simulink model "Copy_of_Qrotor_sim2"  (R2016a)
settings: Solver=ode4  StartTime=0.0  StopTime=T  FixedStep=0.001  RelTol=1e-3
values from neighbouring files (symbols this model uses):
  g = 9.81    [Sim_params.m]
  Ixx = 0.002100    (= 0.0021)    [Drone_params.m]
  Iyy = 0.002417    [Drone_params.m]
  Izz = 0.004633    [Drone_params.m]
  k_learn = 0.000001    (= 1e-06)    [Control_params.m]
  Ki = 3    [Control_params.m]
  KM_1 = KM_GENERAL    (= 0.00509)    [Drone_params.m]
  KM_2 = KM_GENERAL    (= 0.00509)    [Drone_params.m]
  KM_3 = KM_GENERAL    (= 0.00509)    [Drone_params.m]
  KM_4 = KM_GENERAL    (= 0.00509)    [Drone_params.m]
  KM_GENERAL = 0.00509    [Drone_params.m]
  KM_T_1 = KM_T_GENERAL    (= 5e-06)    [Drone_params.m]
  KM_T_2 = KM_T_GENERAL    (= 5e-06)    [Drone_params.m]
  KM_T_3 = KM_T_GENERAL    (= 5e-06)    [Drone_params.m]
  KM_T_4 = KM_T_GENERAL    (= 5e-06)    [Drone_params.m]
  KM_T_GENERAL = 0.000005    (= 5e-06)    [Drone_params.m]
  Kp = Ixx * Ki    [Control_params.m]
  KpP = 5    [Control_params.m]
  m = 0.475    [Drone_params.m]
  n_freq = 0.5    [Sim_params.m]
  PWM_CUT = 1000    [Drone_params.m]
  Tau_1 = Tau    (= 0.1)    [Drone_params.m]
  Tau_2 = Tau    (= 0.1)    [Drone_params.m]
  Tau_3 = Tau    (= 0.1)    [Drone_params.m]
  Tau_4 = Tau    (= 0.1)    [Drone_params.m]
  wnd_amp_p = .1    (= 0.1)    [Wind_params.m]
  wnd_amp_q = 0    [Wind_params.m]
  wnd_amp_r = 0    [Wind_params.m]
  wnd_amp_x = .1    (= 0.1)    [Wind_params.m]
  wnd_amp_y = .1    (= 0.1)    [Wind_params.m]
  wnd_amp_z = .1    (= 0.1)    [Wind_params.m]
  wnd_end_p = 20    [Wind_params.m]
  wnd_end_q = 15    [Wind_params.m]
  wnd_end_r = 15    [Wind_params.m]
  wnd_end_x = 44    [Wind_params.m]
  wnd_end_y = 31    [Wind_params.m]
  wnd_end_z = 49    [Wind_params.m]
  wnd_pqr_enable = 0    [Sim_params.m]
  wnd_ramp_p = 2*pi    (= 6.28318530718)    [Wind_params.m]
  wnd_ramp_q = 0.2    [Wind_params.m]
  wnd_ramp_r = 0.2    [Wind_params.m]
  wnd_ramp_x = .3    (= 0.3)    [Wind_params.m]
  wnd_ramp_y = .3    (= 0.3)    [Wind_params.m]
  wnd_ramp_z = .3    (= 0.3)    [Wind_params.m]
  wnd_start_p = 2    [Wind_params.m]
  wnd_start_q = 2    [Wind_params.m]
  wnd_start_r = 2    [Wind_params.m]
  wnd_start_x = 8    [Wind_params.m]
  wnd_start_y = 3    [Wind_params.m]
  wnd_start_z = 11    [Wind_params.m]
  wnd_xyz_enable = 0    [Sim_params.m]
  X_length = 0.155    [Drone_params.m]
  Y_length = 0.200    (= 0.2)    [Drone_params.m]
undefined symbols (not defined in the file or in its folder): X, Y, Z
libraries: simulink x12, sm_lib x10, nesl_utility x10
(part 1 of 2)
settings Model: Creator=Jet  LastModifiedBy=Jet

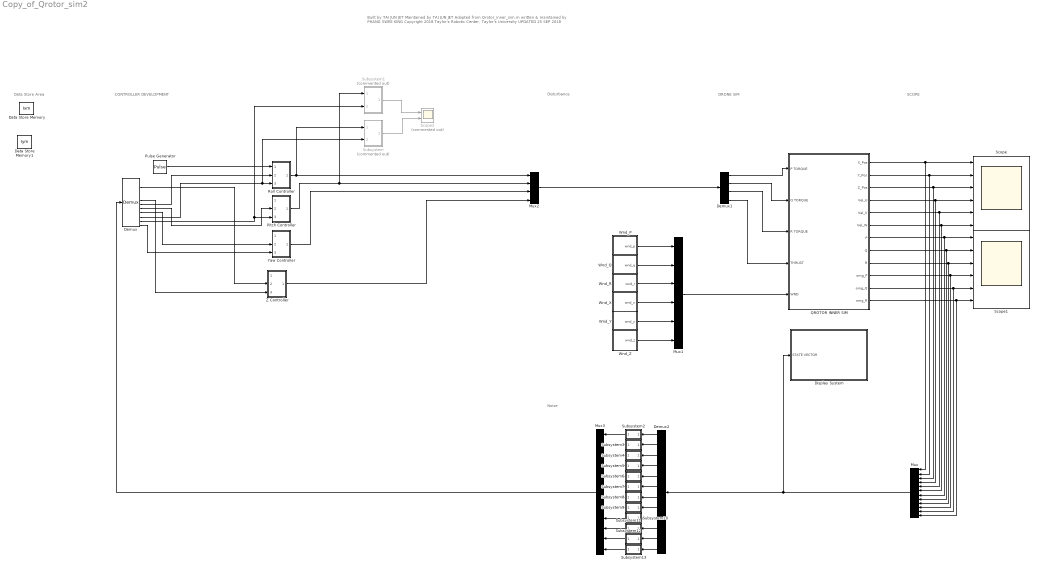
== system Copy_of_Qrotor_sim2 ==
  note: Noise
  note: Data Store Area
  note: Disturbance
  note: SCOPE
  note: DRONE SIM
  note: CONTROLLER DEVELOPMENT
  note: Built by TAI JUN JET
      | Maintained by TAI JUN JET
      | Adopted from Qrotor_inner_sim.m written & maintained by PHANG SWEE KING
      | Copyright 2018 Taylor's Robotic Center, Taylor's University
      | UPDATED 25 SEP 2018
  Data Store Memory : DataStoreMemory  DataStoreName=Ixm  ReadBeforeWriteMsg=warning  WriteAfterWriteMsg=warning  WriteAfterReadMsg=warning  InitialValue=Ixm  ShowAdditionalParam=off  OutDataTypeStr=double
  Data Store Memory1 : DataStoreMemory  DataStoreName=Iym  ReadBeforeWriteMsg=warning  WriteAfterWriteMsg=warning  WriteAfterReadMsg=warning  InitialValue=Iym  ShowAdditionalParam=off  OutDataTypeStr=double
  Demux : Demux  Outputs=12
  Demux1 : Demux
  Demux2 : Demux  Outputs=12
  Display System : Subsystem
  Mux : Mux  Inputs=12
  Mux1 : Mux  Inputs=6
  Mux2 : Mux
  Mux3 : Mux  Inputs=12
  Pitch Controller : Subsystem
  Pulse Generator : DiscretePulseGenerator  PulseType=Time based  Period=11  PulseWidth=50
  "QROTOR INNER SIM " : Subsystem
  "Roll Controller " : Subsystem
  Scope : Scope  NumInputPorts=6
  Scope1 : Scope  NumInputPorts=6
  Scope2 : Scope  Commented=on  NumInputPorts=2
  Subsystem : Subsystem  Commented=on
  Subsystem1 : Subsystem  Commented=on
  Subsystem10 : Subsystem
  Subsystem11 : Subsystem
  Subsystem12 : Subsystem
  Subsystem13 : Subsystem
  Subsystem2 : Subsystem
  Subsystem3 : Subsystem
  Subsystem4 : Subsystem
  Subsystem5 : Subsystem
  Subsystem6 : Subsystem
  Subsystem7 : Subsystem
  Subsystem8 : Subsystem
  Subsystem9 : Subsystem
  Wnd_P : Subsystem
  Wnd_Q : Subsystem
  Wnd_R : Subsystem
  Wnd_X : Subsystem
  Wnd_Y : Subsystem
  Wnd_Z : Subsystem
  Yaw Controller : Subsystem
  "Z Controller " : Subsystem
  wires:
  Mux/1 -> Display System/1(STATE VECTOR), Demux2/1
  Demux/10 -> Subsystem/2(In3), "Roll Controller "/3(In3)
  "QROTOR INNER SIM "/7(P) -> Scope1/1, Mux/7
  "QROTOR INNER SIM "/9(R) -> Scope1/3, Mux/9
  "QROTOR INNER SIM "/2(Y_Pos) -> Scope/2, Mux/2
  "QROTOR INNER SIM "/6(Vel_W) -> Scope/6, Mux/6
  "QROTOR INNER SIM "/11(omg_Q) -> Scope1/5, Mux/11
  "QROTOR INNER SIM "/12(omg_R) -> Scope1/6, Mux/12
  "QROTOR INNER SIM "/1(X_Pos) -> Scope/1, Mux/1
  "QROTOR INNER SIM "/10(omg_P) -> Scope1/4, Mux/10
  "QROTOR INNER SIM "/5(Vel_V) -> Scope/5, Mux/5
  "QROTOR INNER SIM "/8(Q) -> Scope1/2, Mux/8
  "QROTOR INNER SIM "/4(Vel_U) -> Scope/4, Mux/4
  "QROTOR INNER SIM "/3(Z_Pos) -> Scope/3, Mux/3
  Wnd_P/1(wnd_p) -> Mux1/1
  Wnd_Q/1(wnd_q) -> Mux1/2
  Wnd_R/1("wnd_r ") -> Mux1/3
  Wnd_X/1(wnd_x) -> Mux1/4
  Wnd_Y/1(wnd_y) -> Mux1/5
  Wnd_Z/1(wnd_z) -> Mux1/6
  "Roll Controller "/1(Out1) -> Subsystem/1(In2), Mux2/1
  Yaw Controller/1(Out1) -> Mux2/3
  Mux2/1 -> Demux1/1
  Demux1/1 -> "QROTOR INNER SIM "/1(P TORQUE)
  Demux1/2 -> "QROTOR INNER SIM "/2(Q TORQUE)
  Demux1/3 -> "QROTOR INNER SIM "/3(R TORQUE)
  Demux1/4 -> "QROTOR INNER SIM "/4(THRUST)
  Mux1/1 -> "QROTOR INNER SIM "/5(WND)
  Demux/3 -> "Z Controller "/2(In2)
  Demux/6 -> "Z Controller "/3(In3)
  "Z Controller "/1(Out1) -> Mux2/4
  Demux/11 -> Pitch Controller/3(In3), Subsystem1/2(In3)
  Pitch Controller/1(Out1) -> Subsystem1/1(In2), Mux2/2
  Subsystem1/1(Ixm) -> Scope2/1
  Subsystem/1(Iym) -> Scope2/2
  Pulse Generator/1 -> "Roll Controller "/1(In1)
  Demux/8 -> Pitch Controller/2(In2)
  Demux/9 -> Yaw Controller/2(In2)
  Demux/12 -> Yaw Controller/3(In3)
  Demux2/1 -> Subsystem2/1(In1)
  Demux2/2 -> Subsystem3/1(In1)
  Demux2/3 -> Subsystem4/1(In1)
  Demux2/4 -> Subsystem5/1(In1)
  Demux2/5 -> Subsystem6/1(In1)
  Demux2/6 -> Subsystem7/1(In1)
  Demux2/7 -> Subsystem8/1(In1)
  Demux2/8 -> Subsystem9/1(In1)
  Demux2/9 -> Subsystem10/1(In1)
  Demux2/10 -> Subsystem11/1(In1)
  Demux2/11 -> Subsystem12/1(In1)
  Demux2/12 -> Subsystem13/1(In1)
  Subsystem2/1(Out1) -> Mux3/1
  Subsystem3/1(Out1) -> Mux3/2
  Subsystem4/1(Out1) -> Mux3/3
  Subsystem5/1(Out1) -> Mux3/4
  Subsystem6/1(Out1) -> Mux3/5
  Subsystem7/1(Out1) -> Mux3/6
  Subsystem8/1(Out1) -> Mux3/7
  Subsystem9/1(Out1) -> Mux3/8
  Subsystem10/1(Out1) -> Mux3/9
  Subsystem11/1(Out1) -> Mux3/10
  Subsystem12/1(Out1) -> Mux3/11
  Subsystem13/1(Out1) -> Mux3/12
  Mux3/1 -> Demux/1
  Demux/7 -> "Roll Controller "/2(In2)

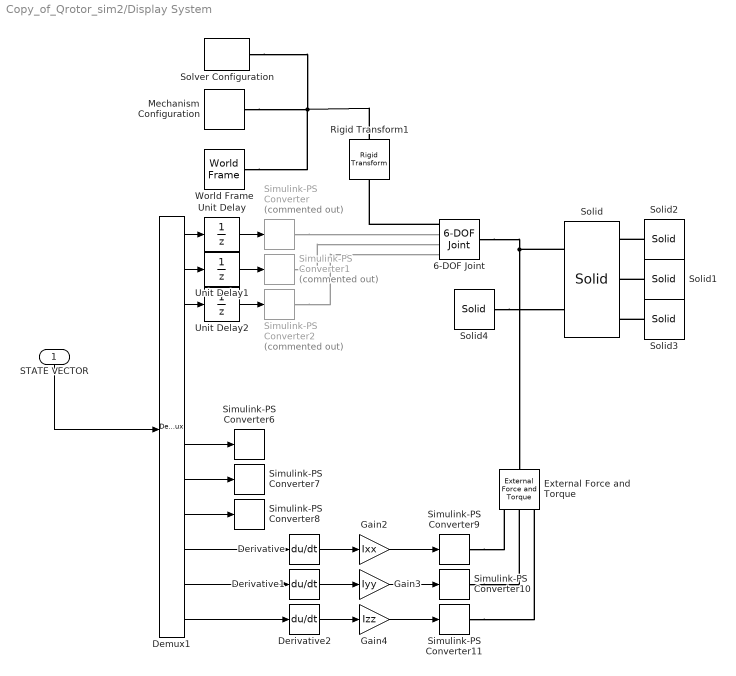
== system Copy_of_Qrotor_sim2/Display System ==
  STATE VECTOR : Inport
  6-DOF Joint : sm_lib/Joints/6-DOF Joint  SenseConstraintForce=off  SenseConstraintForceX=off  SenseConstraintForceY=off  SenseConstraintForceZ=off  SenseConstraintTorque=off  SenseConstraintTorqueX=off  SenseConstraintTorqueY=off  SenseConstraintTorqueZ=off  SenseTotalForce=off  SenseTotalForceX=off  SenseTotalForceY=off  SenseTotalForceZ=off  SenseTotalTorque=off  SenseTotalTorqueX=off  SenseTotalTorqueY=off  SenseTotalTorqueZ=off  CompositeWrenchDir=FollowerOnBase  CompositeWrenchFrame=BaseFrame  PxEquilibriumPosition=0  PxEquilibriumPositionUnits=m  PxSpringStiffness=0  PxSpringStiffnessUnits=N/m  PxDampingCoefficient=0  PxDampingCoefficientUnits=N/(m/s)  PxTorqueActuationMode=ComputedTorque  PxMotionActuationMode=InputMotion  PxSensePosition=off  PxSenseVelocity=off  PxSenseAcceleration=off  PxSenseTorqueForce=off  PxPositionTargetSpecify=on  PxPositionTargetPriority=High  PxPositionTargetValue=0  PxPositionTargetValueUnits=m  PxVelocityTargetSpecify=on  PxVelocityTargetPriority=High  PxVelocityTargetValue=0  PxVelocityTargetValueUnits=m/s  PyEquilibriumPosition=0  PyEquilibriumPositionUnits=m  PySpringStiffness=0  PySpringStiffnessUnits=N/m  PyDampingCoefficient=0  PyDampingCoefficientUnits=N/(m/s)  PyTorqueActuationMode=ComputedTorque  PyMotionActuationMode=InputMotion  PySensePosition=off  PySenseVelocity=off  PySenseAcceleration=off  PySenseTorqueForce=off  PyPositionTargetSpecify=on  PyPositionTargetPriority=High  PyPositionTargetValue=0  PyPositionTargetValueUnits=m  PyVelocityTargetSpecify=on  PyVelocityTargetPriority=High  PyVelocityTargetValue=0  PyVelocityTargetValueUnits=m/s  PzEquilibriumPosition=0  PzEquilibriumPositionUnits=m  PzSpringStiffness=0  PzSpringStiffnessUnits=N/m  PzDampingCoefficient=0  PzDampingCoefficientUnits=N/(m/s)  PzTorqueActuationMode=ComputedTorque  PzMotionActuationMode=InputMotion  PzSensePosition=off  PzSenseVelocity=off  PzSenseAcceleration=off  PzSenseTorqueForce=off  PzPositionTargetSpecify=on  PzPositionTargetPriority=High  PzPositionTargetValue=0  PzPositionTargetValueUnits=m  PzVelocityTargetSpecify=on  PzVelocityTargetPriority=High  PzVelocityTargetValue=0  PzVelocityTargetValueUnits=m/s  SphDefPosRotationMethod=None  SphDefPosRotationAngleUnits=deg  SphDefPosRotationStandardAxis=+Z  SphDefPosRotationAngle=0.0  SphDefPosRotationArbitraryAxis=[0 0 1]  SphDefPosFollAlignAxisA=+X  SphDefPosBaseAlignAxisA=+Y  SphDefPosFollAlignAxisB=+Y  SphDefPosBaseAlignAxisB=+Z  SphDefPosRotationSequenceAxes=FollowerAxes  SphDefPosRotationSequence=XYX  SphDefPosRotationSequenceAngles=[0 0 0]  SphDefPosRotationSequenceAnglesUnits=deg  SphDefPosRotationMatrix=[1 0 0; 0 1 0; 0 0 1]  SphEqPosRotationMethod=None  SphEqPosRotationAngleUnits=deg  SphEqPosRotationStandardAxis=+Z  SphEqPosRotationAngle=0.0  SphEqPosRotationArbitraryAxis=[0 0 1]  SphEqPosFollAlignAxisA=+X  SphEqPosBaseAlignAxisA=+Y  SphEqPosFollAlignAxisB=+Y  SphEqPosBaseAlignAxisB=+Z  SphEqPosRotationSequenceAxes=FollowerAxes  SphEqPosRotationSequence=XYX  SphEqPosRotationSequenceAngles=[0 0 0]  SphEqPosRotationSequenceAnglesUnits=deg  SphEqPosRotationMatrix=[1 0 0; 0 1 0; 0 0 1]  SphSpringStiffness=0  SphSpringStiffnessUnits=N*m/deg  SphDampingCoefficient=0  SphDampingCoefficientUnits=N*m/(deg/s)  SphActuateTorqueX=off  SphActuateTorqueY=off  SphActuateTorqueZ=off  SphActuateTorque=off  SphTorqueActuationMode=NoTorque  SphMotionActuationMode=ComputedMotion  SphActuationFrame=BaseFrame  SphSensePosition=off  SphSenseVelocityX=off  SphSenseVelocityY=off  SphSenseVelocityZ=off  SphSenseVelocity=off  SphSenseAccelerationX=off  SphSenseAccelerationY=off  SphSenseAccelerationZ=off  SphSenseAcceleration=off  SphSenseTorqueX=off  SphSenseTorqueY=off  SphSenseTorqueZ=off  SphSenseTorqueForce=off  SphSensingFrame=BaseFrame  SphPositionTargetRotationMethod=None  SphPositionTargetRotationAngleUnits=deg  SphPositionTargetRotationStandardAxis=+Z  SphPositionTargetRotationAngle=0.0  SphPositionTargetRotationArbitraryAxis=[0 0 1]  SphPositionTargetFollAlignAxisA=+X  SphPositionTargetBaseAlignAxisA=+Y  SphPositionTargetFollAlignAxisB=+Y  SphPositionTargetBaseAlignAxisB=+Z  SphPositionTargetRotationSequenceAxes=FollowerAxes  SphPositionTargetRotationSequence=XYX  SphPositionTargetRotationSequenceAngles=[0 0 0]  SphPositionTargetRotationSequenceAnglesUnits=deg  SphPositionTargetRotationMatrix=[1 0 0; 0 1 0; 0 0 1]  SphPositionTargetSpecify=off  SphPositionTargetPriority=High  SphVelocityTargetValue=[0 0 0]  SphVelocityTargetValueUnits=deg/s  SphVelocityTargetSpecify=off  SphVelocityTargetPriority=High  SphVelocityTargetInFollowerFrame=on
  Demux1 : Demux  Outputs=12
  Derivative : Derivative
  Derivative1 : Derivative
  Derivative2 : Derivative
  External Force and Torque : sm_lib/Forces and Torques/External Force and Torque  ForceResolutionFrame=AttachedFrame  EnableForceX=off  EnableForceY=off  EnableForceZ=off  EnableForce=off  TorqueResolutionFrame=AttachedFrame  EnableTorqueX=on  EnableTorqueY=on  EnableTorqueZ=on  EnableTorque=off
  Gain2 : Gain  Gain=Ixx
  Gain3 : Gain  Gain=Iyy
  Gain4 : Gain  Gain=Izz
  Mechanism Configuration : sm_lib/Utilities/Mechanism Configuration  UniformGravity=Constant  GravityVector=[0 0 0]  GravityUnits=m/s^2  LinearizationDelta=0.001
  Rigid Transform1 : sm_lib/Frames and Transforms/Rigid Transform  TranslationMethod=None  TranslationLengthUnit=m  TranslationStandardAxis=+Z  TranslationStandardOffset=0  TranslationCartesianOffset=[0 0 0]  TranslationROffset=0  TranslationROffsetUnits=m  TranslationZOffset=0  TranslationZOffsetUnits=m  TranslationThetaOffset=0  TranslationThetaOffsetUnits=deg  RotationMethod=AlignedAxes  RotationAngleUnits=deg  RotationStandardAxis=+Z  RotationAngle=0.0  RotationArbitraryAxis=[0 0 1]  FollAlignAxisA=+X  BaseAlignAxisA=+X  FollAlignAxisB=-Z  BaseAlignAxisB=+Z  RotationSequenceAxes=FollowerAxes  RotationSequence=XYX  RotationSequenceAngles=[0 0 0]  RotationSequenceAnglesUnits=deg  RotationMatrix=[1 0 0; 0 1 0; 0 0 1]
  Simulink-PS Converter : nesl_utility/Simulink-PS Converter  Commented=on  PhysicalDomain=network_engine_domain  SubClassName=ps_input  LeftPortType=input  RightPortType=output  PseudoPeriodic=off  Frequencies=[]  NoiseDistribution=none  NoiseParameters=[]  Unit=1  AffineConversion=off  InputFiltering=off  SimscapeFilterOrder=2  InputFilterTimeConstant=0.001  UdotUserProvided=1
  Simulink-PS Converter1 : nesl_utility/Simulink-PS Converter  Commented=on  PhysicalDomain=network_engine_domain  SubClassName=ps_input  LeftPortType=input  RightPortType=output  PseudoPeriodic=off  Frequencies=[]  NoiseDistribution=none  NoiseParameters=[]  Unit=1  AffineConversion=off  InputFiltering=off  SimscapeFilterOrder=2  InputFilterTimeConstant=0.001  UdotUserProvided=1
  Simulink-PS Converter{6..11} (6 alike) : nesl_utility/Simulink-PS Converter  PhysicalDomain=network_engine_domain  SubClassName=ps_input  LeftPortType=input  RightPortType=output  PseudoPeriodic=off  Frequencies=[]  NoiseDistribution=none  NoiseParameters=[]  Unit=1  AffineConversion=off  InputFiltering=off  SimscapeFilterOrder=1  InputFilterTimeConstant=0.001  UdotUserProvided=1
  Simulink-PS Converter2 : nesl_utility/Simulink-PS Converter  Commented=on  PhysicalDomain=network_engine_domain  SubClassName=ps_input  LeftPortType=input  RightPortType=output  PseudoPeriodic=off  Frequencies=[]  NoiseDistribution=none  NoiseParameters=[]  Unit=1  AffineConversion=off  InputFiltering=off  SimscapeFilterOrder=2  InputFilterTimeConstant=0.001  UdotUserProvided=1
  Solid : sm_lib/Body Elements/Solid  InertiaType=Custom  Mass=1  MassUnits=kg  CenterOfMass=[0 0 0]  CenterOfMassUnits=m  MomentsOfInertia=[Ixx Iyy Izz]  MomentsOfInertiaUnits=kg*m^2  ProductsOfInertia=[0 0 0]  ProductsOfInertiaUnits=kg*m^2  DensityBased=on  Density=1000  DensityUnits=kg/(m^3)  DoExposeReferenceFrame=on  SerializedFrames=<Frames><Frame><Id>Frame1</Id><Value><Name>F1</Name><Origin><Source>GeometricFeature</Source><FeatureName>+x -y -z point</FeatureName></Origin><PrimaryAxis><DefinedDirection>+Z</DefinedDirection><Source>ReferenceFrame</Source><SourceDirection>+Z</SourceDirection><FeatureName></FeatureName></PrimaryAxis><SecondaryAxis><DefinedDirection>+X</DefinedDirection><Source>ReferenceFrame</Source><SourceDirection>+X</SourceDirection><FeatureName></FeatureName></SecondaryAxis></Value></Frame><Frame><Id>Frame2</Id><Value><Name>F2</Name><Origin><Source>GeometricFeature</Source><FeatureName>+x +y -z point</FeatureName></Origin><PrimaryAxis><DefinedDirection>+Z</DefinedDirection><Source>ReferenceFrame</Source><SourceDirection>+Z</SourceDirection><FeatureName></FeatureName></PrimaryAxis><SecondaryAxis><DefinedDirection>+X</DefinedDirection><Source>ReferenceFrame</Source><SourceDirection>+X</SourceDirection><FeatureName></FeatureName></SecondaryAxis></Value></Frame><Frame><Id>Frame3</Id><Value><Name>F3</Name><Origin><Source>GeometricFeature</Source><FeatureName>-x -y -z point</FeatureName></Origin><PrimaryAxis><DefinedDirection>+Z</DefinedDirection><Source>ReferenceFrame</Source><SourceDirection>+Z</SourceDirection><FeatureName></FeatureName></PrimaryAxis><SecondaryAxis><DefinedDirection>+X</DefinedDirection><Source>ReferenceFrame</Source><SourceDirection>+X</SourceDirection><FeatureName></FeatureName></SecondaryAxis></Value></Frame><Frame><Id>Frame4</Id><Value><Name>F4</Name><Origin><Source>GeometricFeature</Source><FeatureName>-x +y -z point</FeatureName></Origin><PrimaryAxis><DefinedDirection>+Z</DefinedDirection><Source>ReferenceFrame</Source><SourceDirection>+Z</SourceDirection><FeatureName></FeatureName></PrimaryAxis><SecondaryAxis><DefinedDirection>+X</DefinedDirection><Source>ReferenceFrame</Source><SourceDirection>+X</SourceDirection><FeatureName></FeatureName></SecondaryAxis></Value></Frame></Frames>  GraphicType=FromGeometry  MarkerShape=Sphere  MarkerSize=10  GraphicVisPropType=SimpleVisualProperties  GraphicDiffuseColor=[1 0 0]  GraphicSpecularColor=[1 0.2 0 1.0]  GraphicAmbientColor=[1 .2 0 1.0]  GraphicEmissiveColor=[1 0.0 0.0 1.0]  GraphicShininess=0  GraphicOpacity=1  GeometryShape=Brick  RectangleSize=[1 1]  RectangleSizeUnits=m  BrickDimensions=[Y_length X_length X_length/3]  BrickDimensionUnits=m  CylinderRadius=1  CylinderRadiusUnits=m  CylinderLength=1  CylinderLengthUnits=m  SphereRadius=1  SphereRadiusUnits=m  EllipsoidRadii=[1 1 1]  EllipsoidRadiiUnits=m  ExtrusionCrossSection=[1 1; -1 1; -1 -1; 1 -1]  ExtrusionCrossSectionUnits=m  ExtrusionLength=1  ExtrusionLengthUnits=m  PolygonNumSides=3  PolygonOuterRadius=1  PolygonOuterRadiusUnits=m  ExtGeomFileType=STEP  ExtGeomFileUnits=m  RevolutionCrossSection=[1 1; 1 -1; 2 -1; 2 1]  RevolutionCrossSectionUnits=m  RevolutionExtent=Full  RevolutionAngle=180  RevolutionAngleUnits=deg
  Solid{1..4} (4 alike) : sm_lib/Body Elements/Solid  InertiaType=CalculateFromGeometry  Mass=1  MassUnits=kg  CenterOfMass=[0 0 0]  CenterOfMassUnits=m  MomentsOfInertia=[1 1 1]  MomentsOfInertiaUnits=kg*m^2  ProductsOfInertia=[0 0 0]  ProductsOfInertiaUnits=kg*m^2  DensityBased=on  Density=0  DensityUnits=kg/(m^3)  DoExposeReferenceFrame=on  SerializedFrames=<Frames/>  GraphicType=FromGeometry  MarkerShape=Sphere  MarkerSize=10  GraphicVisPropType=SimpleVisualProperties  GraphicDiffuseColor=[0.5 0.5 0.5]  GraphicSpecularColor=[0.5 0.5 0.5 1.0]  GraphicAmbientColor=[0.15 0.15 0.15 1.0]  GraphicEmissiveColor=[0.0 0.0 0.0 1.0]  GraphicShininess=75  GraphicOpacity=.2  GeometryShape=Cylinder  RectangleSize=[1 1]  RectangleSizeUnits=m  BrickDimensions=[.1 .1 .1]  BrickDimensionUnits=m  CylinderRadius=X_length*Y_length*2  CylinderRadiusUnits=m  CylinderLength=X_length*0.02  CylinderLengthUnits=m  SphereRadius=1  SphereRadiusUnits=m  EllipsoidRadii=[1 1 1]  EllipsoidRadiiUnits=m  ExtrusionCrossSection=[1 1; -1 1; -1 -1; 1 -1]  ExtrusionCrossSectionUnits=m  ExtrusionLength=1  ExtrusionLengthUnits=m  PolygonNumSides=3  PolygonOuterRadius=1  PolygonOuterRadiusUnits=m  ExtGeomFileType=STEP  ExtGeomFileUnits=m  RevolutionCrossSection=[1 1; 1 -1; 2 -1; 2 1]  RevolutionCrossSectionUnits=m  RevolutionExtent=Full  RevolutionAngle=180  RevolutionAngleUnits=deg
  Solver Configuration : nesl_utility/Solver Configuration  PhysicalDomain=network_engine_domain  SubClassName=solver  LeftPortType=input  RightPortType=generic  Accelerate=off  Tones=[]  Harmonics=[]  SimulateNoise=off  Profile=off  UseLocalSampling=off  EnableSwitchedLinearOptims=on  FrequencyDomain=off  UseCCode=off  RelTol=0.001  AbsTol=1e-06  MinStep=1e-09  ToWorkspace=off  RevertToSquareIcSolve=off  NumHomotopyIterations=100  PhasorMode=off  PhasorModeNumHarmonics=1  OverrideAbsTol=off  DoDC=off  ResidualTolerance=1e-09  UseLocalSolver=off  LocalSolverChoice=NE_BACKWARD_EULER_ADVANCER  LocalSolverSampleTime=0.001  DoFixedCost=off  MaxNonlinIter=3  MaxModeIter=2  LinearAlgebra=Sparse  DelaysMemoryBudget=1024  AutomaticFiltering=on  FilteringTimeConstant=0.001
  Unit Delay : UnitDelay  SampleTime=-1
  Unit Delay1 : UnitDelay  SampleTime=-1
  Unit Delay2 : UnitDelay  SampleTime=-1
  World Frame : sm_lib/Frames and Transforms/World Frame
  wires:
  Demux1/2 -> Unit Delay1/1
  Demux1/1 -> Unit Delay/1
  Demux1/3 -> Unit Delay2/1
  Demux1/7 -> Simulink-PS Converter6/1
  Demux1/8 -> Simulink-PS Converter7/1
  Unit Delay/1 -> Simulink-PS Converter/1
  Demux1/12 -> Derivative2/1
  Demux1/10 -> Derivative/1
  Derivative2/1 -> Gain4/1
  Derivative/1 -> Gain2/1
  Demux1/11 -> Derivative1/1
  Unit Delay2/1 -> Simulink-PS Converter2/1
  Gain2/1 -> Simulink-PS Converter9/1
  Gain4/1 -> Simulink-PS Converter11/1
  Demux1/9 -> Simulink-PS Converter8/1
  Derivative1/1 -> Gain3/1
  Gain3/1 -> Simulink-PS Converter10/1
  Unit Delay1/1 -> Simulink-PS Converter1/1
  STATE VECTOR/1 -> Demux1/1
  connections:
  Solid4/RConn1 -- Solid/RConn2
  Simulink-PS Converter1/RConn1 -- 6-DOF Joint/LConn3
  Simulink-PS Converter9/RConn1 -- External Force and Torque/LConn1
  Simulink-PS Converter2/RConn1 -- 6-DOF Joint/LConn4
  Simulink-PS Converter/RConn1 -- 6-DOF Joint/LConn2
  World Frame/RConn1 -- Rigid Transform1/LConn1 -- Mechanism Configuration/RConn1 -- Solver Configuration/RConn1
  Simulink-PS Converter10/RConn1 -- External Force and Torque/LConn2
  Simulink-PS Converter11/RConn1 -- External Force and Torque/LConn3
  Solid2/RConn1 -- Solid/LConn1
  Solid1/RConn1 -- Solid/LConn2
  Solid3/RConn1 -- Solid/LConn3
  Solid/RConn1 -- 6-DOF Joint/RConn1 -- External Force and Torque/RConn1
  6-DOF Joint/LConn1 -- Rigid Transform1/RConn1

== system Copy_of_Qrotor_sim2/Pitch Controller ==
  In1 : Inport
  In2 : Inport  Port=2
  In3 : Inport  Port=3
  Data Store Read : DataStoreRead  DataStoreName=Ixm
  Gain : Gain  Gain=KpP
  Integrator6 : Integrator
  K1 : Gain  Gain=Ki*Kp
  K2 : Gain  Gain=Ki
  Kp : Gain  Gain=Kp
  Matrix Multiply : Product  Multiplication=Matrix(*)
  Sum : Sum  Inputs=+-
  Sum1 : Sum  Inputs=+-
  Sum2 : Sum  Inputs=++-
  Out1 : Outport
  wires:
  K1/1 -> Integrator6/1
  Sum/1 -> K1/1, Kp/1
  In2/1 -> Sum1/2
  In3/1 -> Sum/2, K2/1
  In1/1 -> Sum1/1
  Sum2/1 -> Out1/1
  Integrator6/1 -> Sum2/1
  Kp/1 -> Sum2/2
  K2/1 -> Matrix Multiply/1
  Matrix Multiply/1 -> Sum2/3
  Data Store Read/1 -> Matrix Multiply/2
  Sum1/1 -> Gain/1
  Gain/1 -> Sum/1

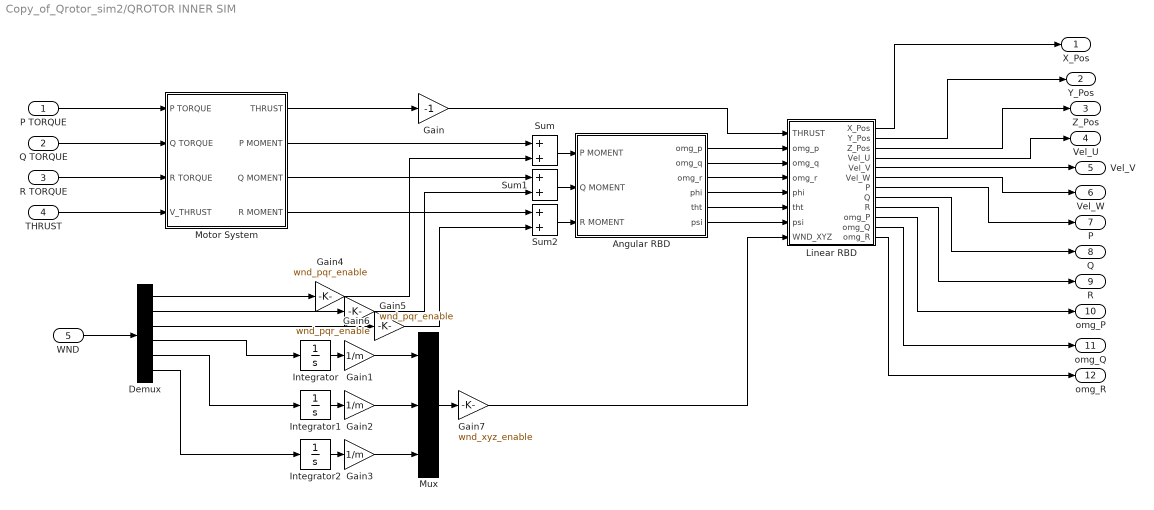
== system Copy_of_Qrotor_sim2/QROTOR INNER SIM  ==
  P TORQUE : Inport
  Q TORQUE : Inport  Port=2
  R TORQUE : Inport  Port=3
  THRUST : Inport  Port=4
  WND : Inport  Port=5
  Angular RBD : Subsystem
  Demux : Demux  Outputs=6
  Gain : Gain  Gain=-1
  Gain1 : Gain  Gain=1/m
  Gain2 : Gain  Gain=1/m
  Gain3 : Gain  Gain=1/m
  Gain4 : Gain  Gain=wnd_pqr_enable
  Gain5 : Gain  Gain=wnd_pqr_enable
  Gain6 : Gain  Gain=wnd_pqr_enable
  Gain7 : Gain  Gain=wnd_xyz_enable
  Integrator : Integrator
  Integrator1 : Integrator
  Integrator2 : Integrator
  Linear RBD : Subsystem
  "Motor System " : Subsystem
  Mux : Mux  Inputs=3
  Sum : Sum
  Sum1 : Sum
  Sum2 : Sum
  X_Pos : Outport
  Y_Pos : Outport  Port=2
  Z_Pos : Outport  Port=3
  Vel_U : Outport  Port=4
  Vel_V : Outport  Port=5
  Vel_W : Outport  Port=6
  P : Outport  Port=7
  Q : Outport  Port=8
  R : Outport  Port=9
  omg_P : Outport  Port=10
  omg_Q : Outport  Port=11
  omg_R : Outport  Port=12
  wires:
  Linear RBD/4(Vel_U) -> Vel_U/1
  Linear RBD/3(Z_Pos) -> Z_Pos/1
  Linear RBD/9(R) -> R/1
  Linear RBD/6(Vel_W) -> Vel_W/1
  Linear RBD/1(X_Pos) -> X_Pos/1
  Linear RBD/7(P) -> P/1
  Linear RBD/2(Y_Pos) -> Y_Pos/1
  Linear RBD/10(omg_P) -> omg_P/1
  Linear RBD/11(omg_Q) -> omg_Q/1
  Linear RBD/12(omg_R) -> omg_R/1
  Linear RBD/8(Q) -> Q/1
  Linear RBD/5(Vel_V) -> Vel_V/1
  Angular RBD/2(omg_q) -> Linear RBD/3(omg_q)
  Angular RBD/4(phi) -> Linear RBD/5(phi)
  Angular RBD/5(tht) -> Linear RBD/6(tht)
  Angular RBD/3(omg_r) -> Linear RBD/4(omg_r)
  Gain/1 -> Linear RBD/1(THRUST)
  Angular RBD/1(omg_p) -> Linear RBD/2(omg_p)
  Angular RBD/6(psi) -> Linear RBD/7(psi)
  THRUST/1 -> "Motor System "/4(V_THRUST)
  P TORQUE/1 -> "Motor System "/1(P TORQUE)
  R TORQUE/1 -> "Motor System "/3(R TORQUE)
  Q TORQUE/1 -> "Motor System "/2(Q TORQUE)
  Sum/1 -> Angular RBD/1(P MOMENT)
  Sum1/1 -> Angular RBD/2(Q MOMENT)
  Sum2/1 -> Angular RBD/3(R MOMENT)
  "Motor System "/2(P MOMENT) -> Sum/1
  "Motor System "/3(Q MOMENT) -> Sum1/1
  "Motor System "/4(R MOMENT) -> Sum2/1
  WND/1 -> Demux/1
  Demux/1 -> Gain4/1
  Demux/2 -> Gain5/1
  Demux/3 -> Gain6/1
  Integrator/1 -> Gain1/1
  Demux/4 -> Integrator/1
  Integrator1/1 -> Gain2/1
  Integrator2/1 -> Gain3/1
  Demux/5 -> Integrator1/1
  Demux/6 -> Integrator2/1
  Gain2/1 -> Mux/2
  Gain1/1 -> Mux/1
  Gain3/1 -> Mux/3
  Mux/1 -> Gain7/1
  Gain4/1 -> Sum/2
  Gain5/1 -> Sum1/2
  Gain6/1 -> Sum2/2
  Gain7/1 -> Linear RBD/8(WND_XYZ)
  "Motor System "/1(THRUST) -> Gain/1

== system Copy_of_Qrotor_sim2/Roll Controller  ==
  In1 : Inport
  In2 : Inport  Port=2
  In3 : Inport  Port=3
  Data Store Read : DataStoreRead  DataStoreName=Ixm
  Gain : Gain  Gain=KpP
  Integrator6 : Integrator
  K1 : Gain  Gain=Ki*Kp
  K2 : Gain  Gain=Ki
  Kp : Gain  Gain=Kp
  Matrix Multiply : Product  Multiplication=Matrix(*)
  Sum : Sum  Inputs=+-
  Sum1 : Sum  Inputs=+-
  Sum2 : Sum  Inputs=++-
  Out1 : Outport
  wires:
  K1/1 -> Integrator6/1
  Sum/1 -> K1/1, Kp/1
  In2/1 -> Sum1/2
  In3/1 -> Sum/2, K2/1
  In1/1 -> Sum1/1
  Sum2/1 -> Out1/1
  Integrator6/1 -> Sum2/1
  Kp/1 -> Sum2/2
  K2/1 -> Matrix Multiply/1
  Matrix Multiply/1 -> Sum2/3
  Data Store Read/1 -> Matrix Multiply/2
  Sum1/1 -> Gain/1
  Gain/1 -> Sum/1

== system Copy_of_Qrotor_sim2/Subsystem ==
  In2 : Inport
  In3 : Inport  Port=2
  Constant : Constant  Value=k_learn
  Data Store Read : DataStoreRead  DataStoreName=Iym
  Data Store Write : DataStoreWrite  DataStoreName=Iym
  Derivative1 : Derivative
  Iym Predictor : MATLAB Function  TreatAsAtomicUnit=on
  Iym : Outport
  wires:
  Data Store Read/1 -> Iym Predictor/4(Iym_sim)
  Iym Predictor/1(Iym_sim_out) -> Iym/1, Data Store Write/1
  Derivative1/1 -> Iym Predictor/1(domg_P)
  In3/1 -> Derivative1/1
  In2/1 -> Iym Predictor/2(p_torque)
  Constant/1 -> Iym Predictor/3(k_learn)

== system Copy_of_Qrotor_sim2/Subsystem1 ==
  In2 : Inport
  In3 : Inport  Port=2
  Constant : Constant  Value=k_learn
  Data Store Read : DataStoreRead  DataStoreName=Ixm
  Data Store Write : DataStoreWrite  DataStoreName=Ixm
  Derivative1 : Derivative
  Ixm Predictor : MATLAB Function  TreatAsAtomicUnit=on
  Ixm : Outport
  wires:
  Data Store Read/1 -> Ixm Predictor/4(Ixm_sim)
  Derivative1/1 -> Ixm Predictor/1(domg_P)
  In3/1 -> Derivative1/1
  In2/1 -> Ixm Predictor/2(p_torque)
  Constant/1 -> Ixm Predictor/3(k_learn)
  Ixm Predictor/1(Ixm_sim_out) -> Ixm/1, Data Store Write/1

== system Copy_of_Qrotor_sim2/Subsystem10 ==
  In1 : Inport
  Band-Limited White Noise : simulink/Sources/Band-Limited White Noise  Cov=n_power  Ts=n_freq  seed=[23341]
  Rate Transition : RateTransition
  Sum : Sum
  Out1 : Outport
  wires:
  Sum/1 -> Out1/1
  In1/1 -> Sum/2
  Band-Limited White Noise/1 -> Rate Transition/1
  Rate Transition/1 -> Sum/1

== system Copy_of_Qrotor_sim2/Subsystem11 ==
  In1 : Inport
  Band-Limited White Noise : simulink/Sources/Band-Limited White Noise  Cov=n_power  Ts=n_freq  seed=[23341]
  Rate Transition : RateTransition
  Sum : Sum
  Out1 : Outport
  wires:
  Sum/1 -> Out1/1
  In1/1 -> Sum/2
  Band-Limited White Noise/1 -> Rate Transition/1
  Rate Transition/1 -> Sum/1

== system Copy_of_Qrotor_sim2/Subsystem12 ==
  In1 : Inport
  Band-Limited White Noise : simulink/Sources/Band-Limited White Noise  Cov=n_power  Ts=n_freq  seed=[23341]
  Rate Transition : RateTransition
  Sum : Sum
  Out1 : Outport
  wires:
  Sum/1 -> Out1/1
  In1/1 -> Sum/2
  Band-Limited White Noise/1 -> Rate Transition/1
  Rate Transition/1 -> Sum/1

== system Copy_of_Qrotor_sim2/Subsystem13 ==
  In1 : Inport
  Band-Limited White Noise : simulink/Sources/Band-Limited White Noise  Cov=n_power  Ts=n_freq  seed=[23341]
  Rate Transition : RateTransition
  Sum : Sum
  Out1 : Outport
  wires:
  Sum/1 -> Out1/1
  In1/1 -> Sum/2
  Band-Limited White Noise/1 -> Rate Transition/1
  Rate Transition/1 -> Sum/1

== system Copy_of_Qrotor_sim2/Subsystem2 ==
  In1 : Inport
  Band-Limited White Noise : simulink/Sources/Band-Limited White Noise  Cov=n_power  Ts=n_freq  seed=[23341]
  Rate Transition : RateTransition
  Sum : Sum
  Out1 : Outport
  wires:
  Sum/1 -> Out1/1
  In1/1 -> Sum/2
  Band-Limited White Noise/1 -> Rate Transition/1
  Rate Transition/1 -> Sum/1

== system Copy_of_Qrotor_sim2/Subsystem3 ==
  In1 : Inport
  Band-Limited White Noise : simulink/Sources/Band-Limited White Noise  Cov=n_power  Ts=n_freq  seed=[23341]
  Rate Transition : RateTransition
  Sum : Sum
  Out1 : Outport
  wires:
  Sum/1 -> Out1/1
  In1/1 -> Sum/2
  Band-Limited White Noise/1 -> Rate Transition/1
  Rate Transition/1 -> Sum/1

== system Copy_of_Qrotor_sim2/Subsystem4 ==
  In1 : Inport
  Band-Limited White Noise : simulink/Sources/Band-Limited White Noise  Cov=n_power  Ts=n_freq  seed=[23341]
  Rate Transition : RateTransition
  Sum : Sum
  Out1 : Outport
  wires:
  Sum/1 -> Out1/1
  In1/1 -> Sum/2
  Band-Limited White Noise/1 -> Rate Transition/1
  Rate Transition/1 -> Sum/1

== system Copy_of_Qrotor_sim2/Subsystem5 ==
  In1 : Inport
  Band-Limited White Noise : simulink/Sources/Band-Limited White Noise  Cov=n_power  Ts=n_freq  seed=[23341]
  Rate Transition : RateTransition
  Sum : Sum
  Out1 : Outport
  wires:
  Sum/1 -> Out1/1
  In1/1 -> Sum/2
  Band-Limited White Noise/1 -> Rate Transition/1
  Rate Transition/1 -> Sum/1

== system Copy_of_Qrotor_sim2/Subsystem6 ==
  In1 : Inport
  Band-Limited White Noise : simulink/Sources/Band-Limited White Noise  Cov=n_power  Ts=n_freq  seed=[23341]
  Rate Transition : RateTransition
  Sum : Sum
  Out1 : Outport
  wires:
  Sum/1 -> Out1/1
  In1/1 -> Sum/2
  Band-Limited White Noise/1 -> Rate Transition/1
  Rate Transition/1 -> Sum/1

== system Copy_of_Qrotor_sim2/Subsystem7 ==
  In1 : Inport
  Band-Limited White Noise : simulink/Sources/Band-Limited White Noise  Cov=n_power  Ts=n_freq  seed=[23341]
  Rate Transition : RateTransition
  Sum : Sum
  Out1 : Outport
  wires:
  Sum/1 -> Out1/1
  In1/1 -> Sum/2
  Band-Limited White Noise/1 -> Rate Transition/1
  Rate Transition/1 -> Sum/1

== system Copy_of_Qrotor_sim2/Subsystem8 ==
  In1 : Inport
  Band-Limited White Noise : simulink/Sources/Band-Limited White Noise  Cov=n_power  Ts=n_freq  seed=[23341]
  Rate Transition : RateTransition
  Sum : Sum
  Out1 : Outport
  wires:
  Sum/1 -> Out1/1
  In1/1 -> Sum/2
  Band-Limited White Noise/1 -> Rate Transition/1
  Rate Transition/1 -> Sum/1

== system Copy_of_Qrotor_sim2/Subsystem9 ==
  In1 : Inport
  Band-Limited White Noise : simulink/Sources/Band-Limited White Noise  Cov=n_power  Ts=n_freq  seed=[23341]
  Rate Transition : RateTransition
  Sum : Sum
  Out1 : Outport
  wires:
  Sum/1 -> Out1/1
  In1/1 -> Sum/2
  Band-Limited White Noise/1 -> Rate Transition/1
  Rate Transition/1 -> Sum/1

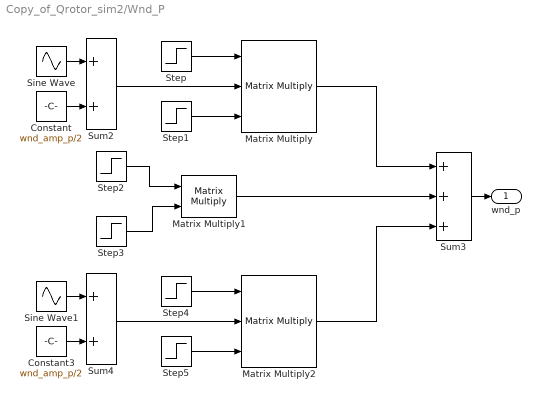
== system Copy_of_Qrotor_sim2/Wnd_P ==
  Constant : Constant  Value=wnd_amp_p/2
  Constant3 : Constant  Value=wnd_amp_p/2
  Matrix Multiply : Product  Inputs=3  Multiplication=Matrix(*)
  Matrix Multiply1 : Product  Multiplication=Matrix(*)
  Matrix Multiply2 : Product  Inputs=3  Multiplication=Matrix(*)
  Sine Wave : Sin  Amplitude=-wnd_amp_p/2  Frequency=wnd_ramp_p  Phase=(pi/2) - (wnd_start_p*wnd_ramp_p)  SampleTime=0
  Sine Wave1 : Sin  Amplitude=wnd_amp_p/2  Frequency=wnd_ramp_p  Phase=-(wnd_end_p*wnd_ramp_p) - pi/2  SampleTime=0
  Step : Step  Time=wnd_start_p  SampleTime=0
  Step1 : Step  Time=wnd_start_p + pi/wnd_ramp_p  Before=1  After=0  SampleTime=0
  Step2 : Step  Time=wnd_start_p + pi/wnd_ramp_p  After=wnd_amp_p  SampleTime=0
  Step3 : Step  Time=(wnd_end_p) - (pi/wnd_ramp_p)  Before=1  After=0  SampleTime=0
  Step4 : Step  Time=wnd_end_p - pi/wnd_ramp_p  SampleTime=0
  Step5 : Step  Time=wnd_end_p  Before=1  After=0  SampleTime=0
  Sum2 : Sum
  Sum3 : Sum  Inputs=+++
  Sum4 : Sum
  wnd_p : Outport
  wires:
  Sine Wave/1 -> Sum2/1
  Constant/1 -> Sum2/2
  Sum2/1 -> Matrix Multiply/2
  Step3/1 -> Matrix Multiply1/2
  Constant3/1 -> Sum4/2
  Sum4/1 -> Matrix Multiply2/2
  Step4/1 -> Matrix Multiply2/1
  Sine Wave1/1 -> Sum4/1
  Step5/1 -> Matrix Multiply2/3
  Matrix Multiply2/1 -> Sum3/3
  Step2/1 -> Matrix Multiply1/1
  Matrix Multiply1/1 -> Sum3/2
  Matrix Multiply/1 -> Sum3/1
  Step/1 -> Matrix Multiply/1
  Step1/1 -> Matrix Multiply/3
  Sum3/1 -> wnd_p/1

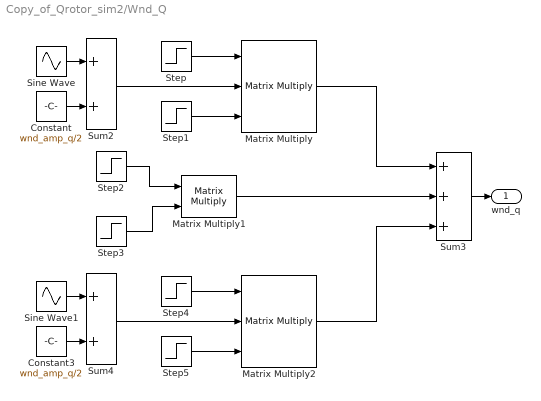
== system Copy_of_Qrotor_sim2/Wnd_Q ==
  Constant : Constant  Value=wnd_amp_q/2
  Constant3 : Constant  Value=wnd_amp_q/2
  Matrix Multiply : Product  Inputs=3  Multiplication=Matrix(*)
  Matrix Multiply1 : Product  Multiplication=Matrix(*)
  Matrix Multiply2 : Product  Inputs=3  Multiplication=Matrix(*)
  Sine Wave : Sin  Amplitude=-wnd_amp_q/2  Frequency=wnd_ramp_q  Phase=(pi/2) - (wnd_start_q*wnd_ramp_q)  SampleTime=0
  Sine Wave1 : Sin  Amplitude=wnd_amp_q/2  Frequency=wnd_ramp_q  Phase=-(wnd_end_q*wnd_ramp_q) - (pi/2)  SampleTime=0
  Step : Step  Time=wnd_start_q  SampleTime=0
  Step1 : Step  Time=wnd_start_q + pi/wnd_ramp_q  Before=1  After=0  SampleTime=0
  Step2 : Step  Time=wnd_start_q + pi/wnd_ramp_q  After=wnd_amp_q  SampleTime=0
  Step3 : Step  Time=(wnd_end_q) - (pi/wnd_ramp_q)  Before=1  After=0  SampleTime=0
  Step4 : Step  Time=wnd_end_q - pi/wnd_ramp_q  SampleTime=0
  Step5 : Step  Time=wnd_end_q  Before=1  After=0  SampleTime=0
  Sum2 : Sum
  Sum3 : Sum  Inputs=+++
  Sum4 : Sum
  wnd_q : Outport
  wires:
  Sum3/1 -> wnd_q/1
  Step1/1 -> Matrix Multiply/3
  Step/1 -> Matrix Multiply/1
  Matrix Multiply/1 -> Sum3/1
  Matrix Multiply1/1 -> Sum3/2
  Step2/1 -> Matrix Multiply1/1
  Matrix Multiply2/1 -> Sum3/3
  Step5/1 -> Matrix Multiply2/3
  Sine Wave1/1 -> Sum4/1
  Step4/1 -> Matrix Multiply2/1
  Sum4/1 -> Matrix Multiply2/2
  Constant3/1 -> Sum4/2
  Step3/1 -> Matrix Multiply1/2
  Sum2/1 -> Matrix Multiply/2
  Constant/1 -> Sum2/2
  Sine Wave/1 -> Sum2/1

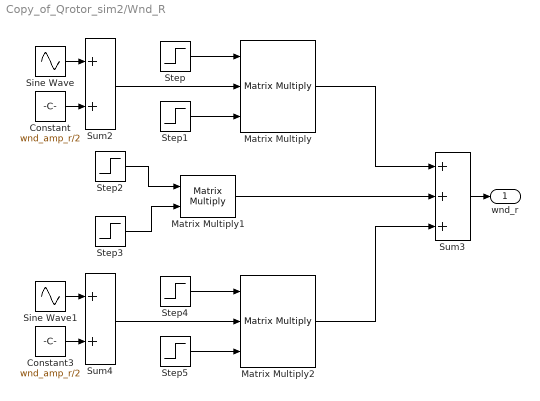
== system Copy_of_Qrotor_sim2/Wnd_R ==
  Constant : Constant  Value=wnd_amp_r/2
  Constant3 : Constant  Value=wnd_amp_r/2
  Matrix Multiply : Product  Inputs=3  Multiplication=Matrix(*)
  Matrix Multiply1 : Product  Multiplication=Matrix(*)
  Matrix Multiply2 : Product  Inputs=3  Multiplication=Matrix(*)
  Sine Wave : Sin  Amplitude=-wnd_amp_r/2  Frequency=wnd_ramp_r  Phase=(pi/2) - (wnd_start_r*wnd_ramp_r)  SampleTime=0
  Sine Wave1 : Sin  Amplitude=wnd_amp_r/2  Frequency=wnd_ramp_r  Phase=-(wnd_end_r*wnd_ramp_r) - (pi/2)  SampleTime=0
  Step : Step  Time=wnd_start_r  SampleTime=0
  Step1 : Step  Time=wnd_start_r + pi/wnd_ramp_r  Before=1  After=0  SampleTime=0
  Step2 : Step  Time=wnd_start_r + pi/wnd_ramp_r  After=wnd_amp_r  SampleTime=0
  Step3 : Step  Time=(wnd_end_r) - (pi/wnd_ramp_r)  Before=1  After=0  SampleTime=0
  Step4 : Step  Time=wnd_end_r - pi/wnd_ramp_r  SampleTime=0
  Step5 : Step  Time=wnd_end_r  Before=1  After=0  SampleTime=0
  Sum2 : Sum
  Sum3 : Sum  Inputs=+++
  Sum4 : Sum
  "wnd_r " : Outport
  wires:
  Sum3/1 -> "wnd_r "/1
  Step1/1 -> Matrix Multiply/3
  Step/1 -> Matrix Multiply/1
  Matrix Multiply/1 -> Sum3/1
  Matrix Multiply1/1 -> Sum3/2
  Step2/1 -> Matrix Multiply1/1
  Matrix Multiply2/1 -> Sum3/3
  Step5/1 -> Matrix Multiply2/3
  Sine Wave1/1 -> Sum4/1
  Step4/1 -> Matrix Multiply2/1
  Sum4/1 -> Matrix Multiply2/2
  Constant3/1 -> Sum4/2
  Step3/1 -> Matrix Multiply1/2
  Sum2/1 -> Matrix Multiply/2
  Constant/1 -> Sum2/2
  Sine Wave/1 -> Sum2/1

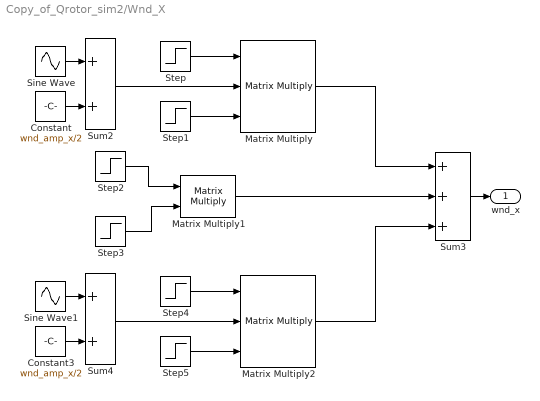
== system Copy_of_Qrotor_sim2/Wnd_X ==
  Constant : Constant  Value=wnd_amp_x/2
  Constant3 : Constant  Value=wnd_amp_x/2
  Matrix Multiply : Product  Inputs=3  Multiplication=Matrix(*)
  Matrix Multiply1 : Product  Multiplication=Matrix(*)
  Matrix Multiply2 : Product  Inputs=3  Multiplication=Matrix(*)
  Sine Wave : Sin  Amplitude=-wnd_amp_x/2  Frequency=wnd_ramp_x  Phase=(pi/2) - (wnd_start_x*wnd_ramp_x)  SampleTime=0
  Sine Wave1 : Sin  Amplitude=wnd_amp_x/2  Frequency=wnd_ramp_x  Phase=-(wnd_end_x*wnd_ramp_x) - pi/2  SampleTime=0
  Step : Step  Time=wnd_start_x  SampleTime=0
  Step1 : Step  Time=wnd_start_x + pi/wnd_ramp_x  Before=1  After=0  SampleTime=0
  Step2 : Step  Time=wnd_start_x + pi/wnd_ramp_x  After=wnd_amp_x  SampleTime=0
  Step3 : Step  Time=(wnd_end_x) - (pi/wnd_ramp_x)  Before=1  After=0  SampleTime=0
  Step4 : Step  Time=wnd_end_x - pi/wnd_ramp_x  SampleTime=0
  Step5 : Step  Time=wnd_end_x  Before=1  After=0  SampleTime=0
  Sum2 : Sum
  Sum3 : Sum  Inputs=+++
  Sum4 : Sum
  wnd_x : Outport
  wires:
  Sine Wave/1 -> Sum2/1
  Constant/1 -> Sum2/2
  Sum2/1 -> Matrix Multiply/2
  Step3/1 -> Matrix Multiply1/2
  Constant3/1 -> Sum4/2
  Sum4/1 -> Matrix Multiply2/2
  Step4/1 -> Matrix Multiply2/1
  Sine Wave1/1 -> Sum4/1
  Step5/1 -> Matrix Multiply2/3
  Matrix Multiply2/1 -> Sum3/3
  Step2/1 -> Matrix Multiply1/1
  Matrix Multiply1/1 -> Sum3/2
  Matrix Multiply/1 -> Sum3/1
  Step/1 -> Matrix Multiply/1
  Step1/1 -> Matrix Multiply/3
  Sum3/1 -> wnd_x/1

== system Copy_of_Qrotor_sim2/Wnd_Y ==
  Constant : Constant  Value=wnd_amp_y/2
  Constant3 : Constant  Value=wnd_amp_y/2
  Matrix Multiply : Product  Inputs=3  Multiplication=Matrix(*)
  Matrix Multiply1 : Product  Multiplication=Matrix(*)
  Matrix Multiply2 : Product  Inputs=3  Multiplication=Matrix(*)
  Sine Wave : Sin  Amplitude=-wnd_amp_y/2  Frequency=wnd_ramp_y  Phase=(pi/2) - (wnd_start_y*wnd_ramp_y)  SampleTime=0
  Sine Wave1 : Sin  Amplitude=wnd_amp_y/2  Frequency=wnd_ramp_y  Phase=-(wnd_end_y*wnd_ramp_y) - (pi/2)  SampleTime=0
  Step : Step  Time=wnd_start_y  SampleTime=0
  Step1 : Step  Time=wnd_start_y + pi/wnd_ramp_y  Before=1  After=0  SampleTime=0
  Step2 : Step  Time=wnd_start_y + pi/wnd_ramp_y  After=wnd_amp_y  SampleTime=0
  Step3 : Step  Time=(wnd_end_y) - (pi/wnd_ramp_y)  Before=1  After=0  SampleTime=0
  Step4 : Step  Time=wnd_end_y - pi/wnd_ramp_y  SampleTime=0
  Step5 : Step  Time=wnd_end_y  Before=1  After=0  SampleTime=0
  Sum2 : Sum
  Sum3 : Sum  Inputs=+++
  Sum4 : Sum
  wnd_y : Outport
  wires:
  Sum3/1 -> wnd_y/1
  Step1/1 -> Matrix Multiply/3
  Step/1 -> Matrix Multiply/1
  Matrix Multiply/1 -> Sum3/1
  Matrix Multiply1/1 -> Sum3/2
  Step2/1 -> Matrix Multiply1/1
  Matrix Multiply2/1 -> Sum3/3
  Step5/1 -> Matrix Multiply2/3
  Sine Wave1/1 -> Sum4/1
  Step4/1 -> Matrix Multiply2/1
  Sum4/1 -> Matrix Multiply2/2
  Constant3/1 -> Sum4/2
  Step3/1 -> Matrix Multiply1/2
  Sum2/1 -> Matrix Multiply/2
  Constant/1 -> Sum2/2
  Sine Wave/1 -> Sum2/1

== system Copy_of_Qrotor_sim2/Wnd_Z ==
  Constant : Constant  Value=wnd_amp_z/2
  Constant3 : Constant  Value=wnd_amp_z/2
  Matrix Multiply : Product  Inputs=3  Multiplication=Matrix(*)
  Matrix Multiply1 : Product  Multiplication=Matrix(*)
  Matrix Multiply2 : Product  Inputs=3  Multiplication=Matrix(*)
  Sine Wave : Sin  Amplitude=-wnd_amp_z/2  Frequency=wnd_ramp_z  Phase=(pi/2) - (wnd_start_z*wnd_ramp_z)  SampleTime=0
  Sine Wave1 : Sin  Amplitude=wnd_amp_z/2  Frequency=wnd_ramp_z  Phase=-(wnd_end_z*wnd_ramp_z) - (pi/2)  SampleTime=0
  Step : Step  Time=wnd_start_z  SampleTime=0
  Step1 : Step  Time=wnd_start_z + pi/wnd_ramp_z  Before=1  After=0  SampleTime=0
  Step2 : Step  Time=wnd_start_z + pi/wnd_ramp_z  After=wnd_amp_z  SampleTime=0
  Step3 : Step  Time=(wnd_end_z) - (pi/wnd_ramp_z)  Before=1  After=0  SampleTime=0
  Step4 : Step  Time=wnd_end_z - pi/wnd_ramp_z  SampleTime=0
  Step5 : Step  Time=wnd_end_z  Before=1  After=0  SampleTime=0
  Sum2 : Sum
  Sum3 : Sum  Inputs=+++
  Sum4 : Sum
  wnd_z : Outport
  wires:
  Sum3/1 -> wnd_z/1
  Step1/1 -> Matrix Multiply/3
  Step/1 -> Matrix Multiply/1
  Matrix Multiply/1 -> Sum3/1
  Matrix Multiply1/1 -> Sum3/2
  Step2/1 -> Matrix Multiply1/1
  Matrix Multiply2/1 -> Sum3/3
  Step5/1 -> Matrix Multiply2/3
  Sine Wave1/1 -> Sum4/1
  Step4/1 -> Matrix Multiply2/1
  Sum4/1 -> Matrix Multiply2/2
  Constant3/1 -> Sum4/2
  Step3/1 -> Matrix Multiply1/2
  Sum2/1 -> Matrix Multiply/2
  Constant/1 -> Sum2/2
  Sine Wave/1 -> Sum2/1

== system Copy_of_Qrotor_sim2/Yaw Controller ==
  In1 : Inport
  In2 : Inport  Port=2
  In3 : Inport  Port=3
  Data Store Read : DataStoreRead  DataStoreName=Ixm
  Gain : Gain  Gain=KpP
  Integrator6 : Integrator
  K1 : Gain  Gain=Ki*Kp
  K2 : Gain  Gain=Ki
  Kp : Gain  Gain=Kp
  Matrix Multiply : Product  Multiplication=Matrix(*)
  Sum : Sum  Inputs=+-
  Sum1 : Sum  Inputs=+-
  Sum2 : Sum  Inputs=++-
  Out1 : Outport
  wires:
  K1/1 -> Integrator6/1
  Sum/1 -> K1/1, Kp/1
  In2/1 -> Sum1/2
  In3/1 -> Sum/2, K2/1
  In1/1 -> Sum1/1
  Sum2/1 -> Out1/1
  Integrator6/1 -> Sum2/1
  Kp/1 -> Sum2/2
  K2/1 -> Matrix Multiply/1
  Matrix Multiply/1 -> Sum2/3
  Data Store Read/1 -> Matrix Multiply/2
  Sum1/1 -> Gain/1
  Gain/1 -> Sum/1

== system Copy_of_Qrotor_sim2/Z Controller  ==
  In1 : Inport
  In2 : Inport  Port=2
  In3 : Inport  Port=3
  Constant : Constant  Value=m*g
  Gain : Gain  Gain=-1
  Gain1 : Gain  Gain=-1
  Integrator6 : Integrator
  K1 : Gain  Gain=Ki*Kp
  K2 : Gain  Gain=Ki*m
  Kp : Gain  Gain=Kp
  Sum : Sum  Inputs=+-
  Sum1 : Sum  Inputs=+-
  Sum2 : Sum  Inputs=++-
  Sum3 : Sum
  Out1 : Outport
  wires:
  K1/1 -> Integrator6/1
  Sum/1 -> K1/1, Kp/1
  In2/1 -> Gain/1
  Sum1/1 -> Sum/1
  In3/1 -> Gain1/1
  In1/1 -> Sum1/1
  Integrator6/1 -> Sum2/1
  Kp/1 -> Sum2/2
  K2/1 -> Sum2/3
  Sum2/1 -> Sum3/1
  Sum3/1 -> Out1/1
  Constant/1 -> Sum3/2
  Gain/1 -> Sum1/2
  Gain1/1 -> Sum/2, K2/1

== system Copy_of_Qrotor_sim2/QROTOR INNER SIM /Angular RBD ==
  P MOMENT : Inport
  Q MOMENT : Inport  Port=2
  R MOMENT : Inport  Port=3
  Integrator3 : Integrator
  Integrator4 : Integrator
  Integrator5 : Integrator
  RBD Angle : Subsystem
  RBD Angular Acce : Subsystem
  RBD Angular Rate : MATLAB Function  TreatAsAtomicUnit=on
  omg_p : Outport
  omg_q : Outport  Port=2
  omg_r : Outport  Port=3
  phi : Outport  Port=4
  tht : Outport  Port=5
  psi : Outport  Port=6
  wires:
  RBD Angular Acce/2(domg_q) -> Integrator4/1
  RBD Angular Acce/3(domg_r) -> Integrator5/1
  RBD Angular Rate/2(tht_dot) -> RBD Angle/2(tht_dot)
  RBD Angular Acce/1(domg_p) -> Integrator3/1
  RBD Angular Rate/3(psi_dot) -> RBD Angle/3(psi_dot)
  RBD Angular Rate/1(phi_dot) -> RBD Angle/1(phi_dot)
  RBD Angle/1(phi) -> phi/1, RBD Angular Rate/4(phi)
  RBD Angle/2(tht) -> tht/1, RBD Angular Rate/5(tht)
  Integrator5/1 -> omg_r/1, RBD Angular Acce/6(omg_r), RBD Angular Rate/3(omg_r)
  RBD Angle/3(psi) -> RBD Angular Rate/6(psi), psi/1
  Integrator3/1 -> omg_p/1, RBD Angular Acce/4(omg_p), RBD Angular Rate/1(omg_p)
  Integrator4/1 -> omg_q/1, RBD Angular Acce/5(omg_q), RBD Angular Rate/2(omg_q)
  P MOMENT/1 -> RBD Angular Acce/1(p_moment)
  Q MOMENT/1 -> RBD Angular Acce/2(q_moment)
  R MOMENT/1 -> RBD Angular Acce/3(r_moment)

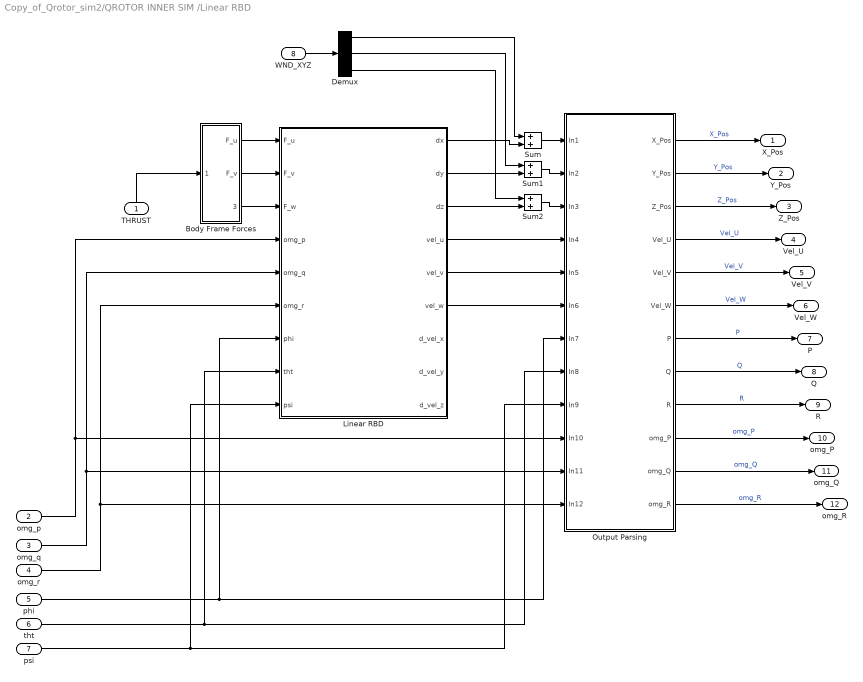
== system Copy_of_Qrotor_sim2/QROTOR INNER SIM /Linear RBD ==
  THRUST : Inport
  omg_p : Inport  Port=2
  omg_q : Inport  Port=3
  omg_r : Inport  Port=4
  phi : Inport  Port=5
  tht : Inport  Port=6
  psi : Inport  Port=7
  WND_XYZ : Inport  Port=8
  Body Frame Forces : Subsystem
  Demux : Demux  Outputs=3
  Linear RBD : Subsystem
  Output Parsing : Subsystem
  Sum : Sum
  Sum1 : Sum
  Sum2 : Sum
  X_Pos : Outport
  Y_Pos : Outport  Port=2
  Z_Pos : Outport  Port=3
  Vel_U : Outport  Port=4
  Vel_V : Outport  Port=5
  Vel_W : Outport  Port=6
  P : Outport  Port=7
  Q : Outport  Port=8
  R : Outport  Port=9
  omg_P : Outport  Port=10
  omg_Q : Outport  Port=11
  omg_R : Outport  Port=12
  wires:
  Output Parsing/12(omg_R) -> omg_R/1  "omg_R"
  Output Parsing/3(Z_Pos) -> Z_Pos/1  "Z_Pos"
  Output Parsing/1(X_Pos) -> X_Pos/1  "X_Pos"
  Output Parsing/11(omg_Q) -> omg_Q/1  "omg_Q"
  Output Parsing/7(P) -> P/1  "P"
  Output Parsing/8(Q) -> Q/1  "Q"
  Output Parsing/5(Vel_V) -> Vel_V/1  "Vel_V"
  Output Parsing/6(Vel_W) -> Vel_W/1  "Vel_W"
  Output Parsing/9(R) -> R/1  "R"
  Output Parsing/10(omg_P) -> omg_P/1  "omg_P"
  Output Parsing/4(Vel_U) -> Vel_U/1  "Vel_U"
  Output Parsing/2(Y_Pos) -> Y_Pos/1  "Y_Pos"
  THRUST/1 -> Body Frame Forces/1("Z_rt ")
  omg_r/1 -> Linear RBD/6(omg_r), Output Parsing/12(In12)
  omg_q/1 -> Linear RBD/5(omg_q), Output Parsing/11(In11)
  omg_p/1 -> Linear RBD/4(omg_p), Output Parsing/10(In10)
  phi/1 -> Linear RBD/7(phi), Output Parsing/7(In7)
  tht/1 -> Output Parsing/8(In8), Linear RBD/8(tht)
  psi/1 -> Output Parsing/9(In9), Linear RBD/9(psi)
  Linear RBD/4(vel_u) -> Output Parsing/4(In4)
  Body Frame Forces/2(F_v) -> Linear RBD/2(F_v)
  Linear RBD/5(vel_v) -> Output Parsing/5(In5)
  Body Frame Forces/3(F_w) -> Linear RBD/3(F_w)
  Body Frame Forces/1(F_u) -> Linear RBD/1(F_u)
  Linear RBD/6(vel_w) -> Output Parsing/6(In6)
  WND_XYZ/1 -> Demux/1
  Sum/1 -> Output Parsing/1(In1)
  Sum1/1 -> Output Parsing/2(In2)
  Sum2/1 -> Output Parsing/3(In3)
  Demux/1 -> Sum/1
  Demux/2 -> Sum1/1
  Demux/3 -> Sum2/1
  Linear RBD/1(dx) -> Sum/2
  Linear RBD/2(dy) -> Sum1/2
  Linear RBD/3(dz) -> Sum2/2

== system Copy_of_Qrotor_sim2/QROTOR INNER SIM /Motor System  ==
  P TORQUE : Inport
  Q TORQUE : Inport  Port=2
  R TORQUE : Inport  Port=3
  V_THRUST : Inport  Port=4
  Body Frame Moments : Subsystem
  Command to Motor Map : Subsystem
  Constant : Constant  Value=PWM_CUT
  Motor Dynamics : Subsystem
  THRUST : Outport
  P MOMENT : Outport  Port=2
  Q MOMENT : Outport  Port=3
  R MOMENT : Outport  Port=4
  wires:
  Motor Dynamics/4(M4_THRUST) -> Body Frame Moments/4(M4_THRUST)
  Motor Dynamics/2(M2_THRUST) -> Body Frame Moments/2(M2_THRUST)
  Motor Dynamics/1(M1_THRUST) -> Body Frame Moments/1(M1_THRUST)
  Motor Dynamics/3(M3_THRUST) -> Body Frame Moments/3(M3_THRUST)
  Command to Motor Map/2(M2_PWM) -> Motor Dynamics/2(M2_PWMIN)
  Command to Motor Map/3(M3_PWM) -> Motor Dynamics/3(M3_PWMIN)
  Command to Motor Map/4(M4_PWM) -> Motor Dynamics/4(M4_PWMIN)
  Constant/1 -> Motor Dynamics/5("PWM_CUTOFF ")
  Body Frame Moments/3(q_moment) -> Q MOMENT/1
  Body Frame Moments/4("r_moment ") -> R MOMENT/1
  Body Frame Moments/1(Thrust_total) -> THRUST/1
  Body Frame Moments/2(p_moment) -> P MOMENT/1
  Q TORQUE/1 -> Command to Motor Map/2(Q_TORQUE)
  R TORQUE/1 -> Command to Motor Map/3(R_TORQUE)
  P TORQUE/1 -> Command to Motor Map/1(P_TORQUE)
  V_THRUST/1 -> Command to Motor Map/4(THRUST)
  Command to Motor Map/1(M1_PWM) -> Motor Dynamics/1(M1_PWMIN)

== system Copy_of_Qrotor_sim2/QROTOR INNER SIM /Angular RBD/RBD Angle ==
  phi_dot : Inport
  tht_dot : Inport  Port=2
  psi_dot : Inport  Port=3
  Integrator : Integrator
  Integrator1 : Integrator
  Integrator2 : Integrator
  phi : Outport
  tht : Outport  Port=2
  psi : Outport  Port=3
  wires:
  tht_dot/1 -> Integrator1/1
  psi_dot/1 -> Integrator2/1
  phi_dot/1 -> Integrator/1
  Integrator/1 -> phi/1
  Integrator1/1 -> tht/1
  Integrator2/1 -> psi/1

== system Copy_of_Qrotor_sim2/QROTOR INNER SIM /Angular RBD/RBD Angular Acce ==
  p_moment : Inport
  q_moment : Inport  Port=2
  r_moment : Inport  Port=3
  omg_p : Inport  Port=4
  omg_q : Inport  Port=5
  omg_r : Inport  Port=6
  AngularRBD_AcceCalc : MATLAB Function  TreatAsAtomicUnit=on
  Constant : Constant  Value=Ixx
  Constant1 : Constant  Value=Iyy
  Constant2 : Constant  Value=Izz
  domg_p : Outport
  domg_q : Outport  Port=2
  domg_r : Outport  Port=3
  wires:
  p_moment/1 -> AngularRBD_AcceCalc/1(M_p)
  q_moment/1 -> AngularRBD_AcceCalc/2(M_q)
  r_moment/1 -> AngularRBD_AcceCalc/3(M_r)
  AngularRBD_AcceCalc/1(domg_p) -> domg_p/1
  AngularRBD_AcceCalc/2(domg_q) -> domg_q/1
  AngularRBD_AcceCalc/3(domg_r) -> domg_r/1
  omg_p/1 -> AngularRBD_AcceCalc/4(omg_p)
  omg_q/1 -> AngularRBD_AcceCalc/5(omg_q)
  omg_r/1 -> AngularRBD_AcceCalc/6(omg_r)
  Constant/1 -> AngularRBD_AcceCalc/7(Ixx)
  Constant1/1 -> AngularRBD_AcceCalc/8(Iyy)
  Constant2/1 -> AngularRBD_AcceCalc/9(Izz)

== system Copy_of_Qrotor_sim2/QROTOR INNER SIM /Linear RBD/Body Frame Forces ==
  "Z_rt " : Inport
  Constant : Constant  Value=0
  Constant1 : Constant  Value=0
  F_u : Outport
  F_v : Outport  Port=2
  F_w : Outport  Port=3
  wires:
  "Z_rt "/1 -> F_w/1
  Constant/1 -> F_u/1
  Constant1/1 -> F_v/1
